simulink library "INT_Diff_PlausPrtTrq"  (R2016b)
settings: Solver=VariableStepAuto  StartTime=0.0  StopTime=10.0  RelTol=1e-3
settings Model: Creator=Administrator  LastModifiedBy=Administrator

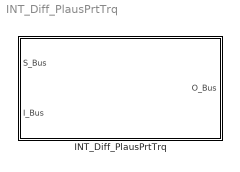
== system INT_Diff_PlausPrtTrq ==
  INT_Diff_PlausPrtTrq : Subsystem

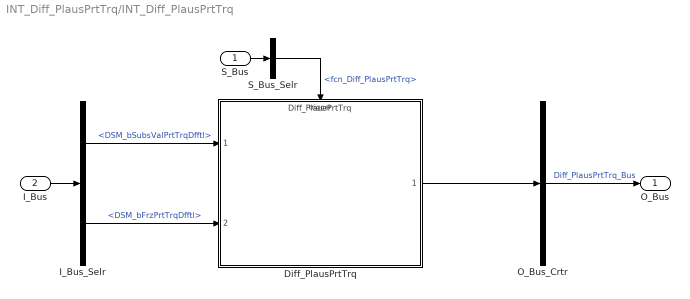
== system INT_Diff_PlausPrtTrq/INT_Diff_PlausPrtTrq ==
  S_Bus : Inport
  I_Bus : Inport  Port=2
  Diff_PlausPrtTrq : ModelReference  ModelNameDialog=Diff_PlausPrtTrq  SimulationMode=Normal  ModelReferenceVersion=1.11  TriggerPortName=function  TriggerPortTriggerType=function-call  TriggerPortStatesWhenEnabling=held
  I_Bus_Selr : BusSelector  OutputSignals=DSM_bSubsValPrtTrqDfftl,DSM_bFrzPrtTrqDfftl
  O_Bus_Crtr : BusCreator  Inputs=1
  S_Bus_Selr : BusSelector  OutputSignals=fcn_Diff_PlausPrtTrq
  O_Bus : Outport
  wires:
  S_Bus_Selr/1 -> Diff_PlausPrtTrq/Trigger  "<fcn_Diff_PlausPrtTrq>"
  S_Bus/1 -> S_Bus_Selr/1
  I_Bus/1 -> I_Bus_Selr/1
  I_Bus_Selr/1 -> Diff_PlausPrtTrq/1  "<DSM_bSubsValPrtTrqDfftl>"
  I_Bus_Selr/2 -> Diff_PlausPrtTrq/2  "<DSM_bFrzPrtTrqDfftl>"
  O_Bus_Crtr/1 -> O_Bus/1  "Diff_PlausPrtTrq_Bus"
  Diff_PlausPrtTrq/1 -> O_Bus_Crtr/1
